simulink model "SecRwLtStFtrstIsPosChk"  (R2024b)
settings: Solver=FixedStepDiscrete  StartTime=0.0  StopTime=10.0  FixedStep=0.01  RelTol=1e-3
undefined symbols (not defined in the file or in its folder): KeSMSuSecRwStFtrstUpwdDnwdPosDelta_Val, KeSMSuSecRwStFtrstUpwdDnwdPosTolr_Val
libraries: StIsPosChkLib x9, simulink x5
settings Model: ModifiedHistory=2023.8.1 V2.0.0 CR401790 增加模式21-26  Creator=sn2xws  LastModifiedBy=sn55gm
settings SolverCC: AlgebraicLoopSolver=TrustRegion
settings DataIOCC: SaveFormat=StructureWithTime  ReturnWorkspaceOutputs=off
settings OptimizationCC: DefaultParameterBehavior=Inlined  EnhancedBackFolding=on  PassReuseOutputArgsAs=Individual arguments  ZeroExternalMemoryAtStartup=off  ZeroInternalMemoryAtStartup=off  OptimizeBlockOrder=speed  DifferentSizesBufferReuse=on  OptimizationCustomize=off  EfficientTunableParamExpr=on
settings DebuggingCC: ParameterTunabilityLossMsg=error  UnconnectedInputMsg=warning  UnconnectedOutputMsg=warning  UnconnectedLineMsg=warning  ArithmeticOperatorsInVariantConditions=warning
settings ModelReferenceCC: EnableRefExpFcnMdlSchedulingChecks=on  ModelReferenceNumInstancesAllowed=Single
settings SFSimCC: MATLABDynamicMemAlloc=off  CustomCodeUndefinedFunction=UseInterfaceOnly
settings RTWCC: Description=AUTOSAR  SystemTargetFile=autosar.tlc  GenCodeOnly=on  TemplateMakefile=ert_default_tmf  GenerateReport=on  IncludeHyperlinkInReport=on  LaunchReport=on  DataTypeReplacement=CDataTypesFixedWidth  GenerateTraceInfo=on  GenerateTraceReport=on  GenerateTraceReportSl=on  GenerateTraceReportSf=on  GenerateTraceReportEml=on  GenerateCodeMetricsReport=on  GPUComputeCapability=3.5
settings CodeAppCC: ForceParamTrailComments=on  IgnoreCustomStorageClasses=off  OperatorAnnotations=on  SimulinkDataObjDesc=on  SFDataObjDesc=on  InsertBlockDesc=on
settings STFCustomTargetCC: TargetLangStandard=C99 (ISO)  MultiwordLength=256  ParMdlRefBuildCompliant=on  CompOptLevelCompliant=on  IncludeMdlTerminateFcn=off  CombineOutputUpdateFcns=on  SuppressErrorStatus=on  ERTCustomFileBanners=on  SupportNonFinite=off  SupportComplex=off  SupportContinuousTime=off  SupportNonInlinedSFcns=off  RemoveResetFunc=on  MATLABClassNameForMDSCustomization=Simulink.SoftwareTarget.ERTCustomization  AutosarCompliant=on  UseToolchainInfoCompliant=on  LookupTableObjectStructAxisOrder=2,1,3,4,...  LUTObjectStructOrderEvenSpacing=Size,Table,Breakpoints  SystemTargetFile=autosar.tlc
settings ERTTargetCC: TargetLangStandard=C99 (ISO)  ConcurrentExecutionCompliant=off  IncludeMdlTerminateFcn=off  SuppressErrorStatus=on  SupportNonFinite=off  SupportComplex=off  ModelStepFunctionPrototypeControlCompliant=off  CPPClassGenCompliant=off  AutosarCompliant=on  LookupTableObjectStructAxisOrder=2,1,3,4,...  LUTObjectStructOrderEvenSpacing=Size,Table,Breakpoints  ERTCustomFileTemplate=example_file_process.tlc  ERTFilePackagingFormat=Compact  BooleanTrueId=TRUE  BooleanFalseId=FALSE  DynamicArrayContainerType=coder::array

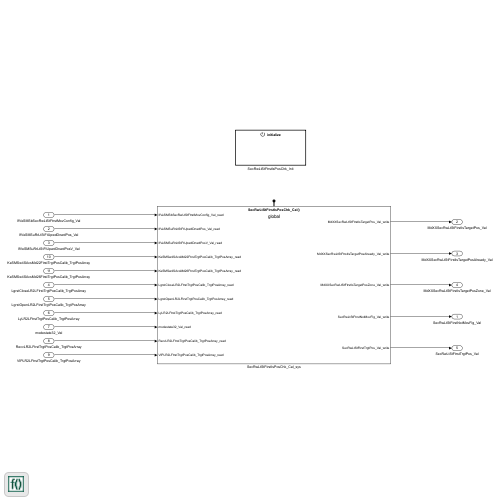
[thumbnail: Simulink's stored preview of the top-level diagram]
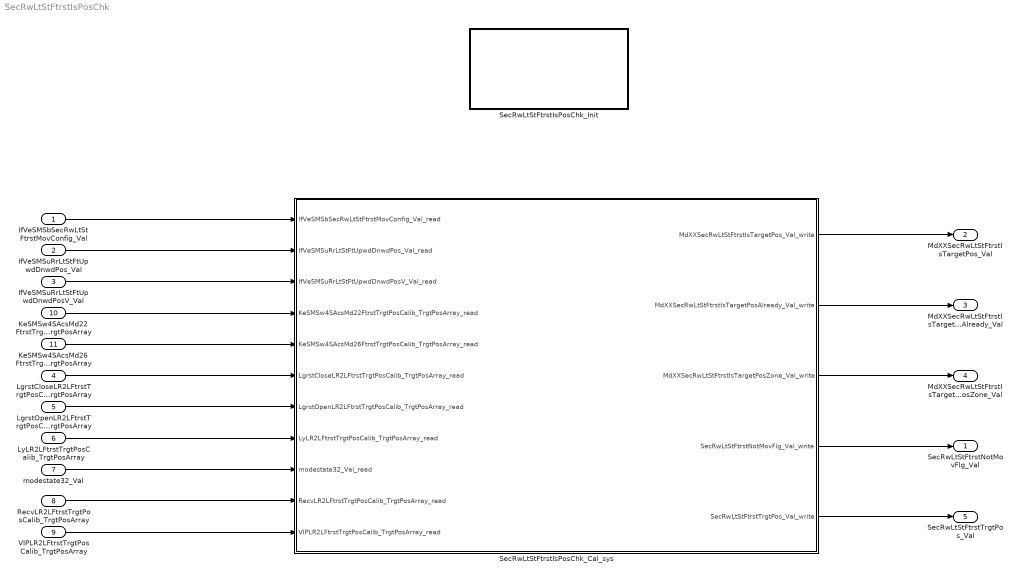
== system SecRwLtStFtrstIsPosChk ==
  IfVeSMSbSecRwLtStFtrstMovConfig_Val : Inport  OutDataTypeStr=boolean  PortDimensions=1
  IfVeSMSuRrLtStFtUpwdDnwdPos_Val : Inport  Port=2  OutDataTypeStr=uint16  PortDimensions=1
  IfVeSMSuRrLtStFtUpwdDnwdPosV_Val : Inport  Port=3  OutDataTypeStr=boolean  PortDimensions=1
  LgrstCloseLR2LFtrstTrgtPosCalib_TrgtPosArray : Inport  Description=|  Port=4  OutDataTypeStr=uint16  PortDimensions=3
      | 0:Pos
      | 1:Max
      | 2:Min
  LgrstOpenLR2LFtrstTrgtPosCalib_TrgtPosArray : Inport  Description=|  Port=5  OutDataTypeStr=uint16  PortDimensions=3
      | 0:Pos
      | 1:Max
      | 2:Min
  LyLR2LFtrstTrgtPosCalib_TrgtPosArray : Inport  Description=|  Port=6  OutDataTypeStr=uint16  PortDimensions=3
      | 0:Pos
      | 1:Max
      | 2:Min
  modestate32_Val : Inport  Port=7  OutDataTypeStr=uint32  PortDimensions=1
  RecvLR2LFtrstTrgtPosCalib_TrgtPosArray : Inport  Description=|  Port=8  OutDataTypeStr=uint16  PortDimensions=3
      | 0:Pos
      | 1:Max
      | 2:Min
  VIPLR2LFtrstTrgtPosCalib_TrgtPosArray : Inport  Description=|  Port=9  OutDataTypeStr=uint16  PortDimensions=3
      | 0:Pos
      | 1:Max
      | 2:Min
  KeSMSw4SAcsMd22FtrstTrgtPosCalib_TrgtPosArray : Inport  Description=|  Port=10  OutDataTypeStr=uint16  PortDimensions=3
      | 0:Pos
      | 1:Max
      | 2:Min
  KeSMSw4SAcsMd26FtrstTrgtPosCalib_TrgtPosArray : Inport  Description=|  Port=11  OutDataTypeStr=uint16  PortDimensions=3
      | 0:Pos
      | 1:Max
      | 2:Min
  SecRwLtStFtrstIsPosChk_Cal_sys : Subsystem
  SecRwLtStFtrstIsPosChk_Init : Subsystem
  SecRwLtStFtrstNotMovFlg_Val : Outport  OutDataTypeStr=boolean  PortDimensions=1  VectorParamsAs1DForOutWhenUnconnected=off
  MdXXSecRwLtStFtrstIsTargetPos_Val : Outport  Port=2  OutDataTypeStr=uint32  PortDimensions=1  VectorParamsAs1DForOutWhenUnconnected=off
  MdXXSecRwLtStFtrstIsTargetPosAlready_Val : Outport  Port=3  OutDataTypeStr=uint32  PortDimensions=1  VectorParamsAs1DForOutWhenUnconnected=off
  MdXXSecRwLtStFtrstIsTargetPosZone_Val : Outport  Port=4  OutDataTypeStr=uint32  PortDimensions=1  VectorParamsAs1DForOutWhenUnconnected=off
  SecRwLtStFtrstTrgtPos_Val : Outport  Port=5  OutDataTypeStr=uint16  PortDimensions=1  VectorParamsAs1DForOutWhenUnconnected=off
  wires:
  IfVeSMSbSecRwLtStFtrstMovConfig_Val/1 -> SecRwLtStFtrstIsPosChk_Cal_sys/1(IfVeSMSbSecRwLtStFtrstMovConfig_Val_read)
  IfVeSMSuRrLtStFtUpwdDnwdPos_Val/1 -> SecRwLtStFtrstIsPosChk_Cal_sys/2(IfVeSMSuRrLtStFtUpwdDnwdPos_Val_read)
  IfVeSMSuRrLtStFtUpwdDnwdPosV_Val/1 -> SecRwLtStFtrstIsPosChk_Cal_sys/3(IfVeSMSuRrLtStFtUpwdDnwdPosV_Val_read)
  LgrstCloseLR2LFtrstTrgtPosCalib_TrgtPosArray/1 -> SecRwLtStFtrstIsPosChk_Cal_sys/6(LgrstCloseLR2LFtrstTrgtPosCalib_TrgtPosArray_read)
  LgrstOpenLR2LFtrstTrgtPosCalib_TrgtPosArray/1 -> SecRwLtStFtrstIsPosChk_Cal_sys/7(LgrstOpenLR2LFtrstTrgtPosCalib_TrgtPosArray_read)
  LyLR2LFtrstTrgtPosCalib_TrgtPosArray/1 -> SecRwLtStFtrstIsPosChk_Cal_sys/8(LyLR2LFtrstTrgtPosCalib_TrgtPosArray_read)
  modestate32_Val/1 -> SecRwLtStFtrstIsPosChk_Cal_sys/9(modestate32_Val_read)
  RecvLR2LFtrstTrgtPosCalib_TrgtPosArray/1 -> SecRwLtStFtrstIsPosChk_Cal_sys/10(RecvLR2LFtrstTrgtPosCalib_TrgtPosArray_read)
  VIPLR2LFtrstTrgtPosCalib_TrgtPosArray/1 -> SecRwLtStFtrstIsPosChk_Cal_sys/11(VIPLR2LFtrstTrgtPosCalib_TrgtPosArray_read)
  SecRwLtStFtrstIsPosChk_Cal_sys/1(MdXXSecRwLtStFtrstIsTargetPos_Val_write) -> MdXXSecRwLtStFtrstIsTargetPos_Val/1
  SecRwLtStFtrstIsPosChk_Cal_sys/2(MdXXSecRwLtStFtrstIsTargetPosAlready_Val_write) -> MdXXSecRwLtStFtrstIsTargetPosAlready_Val/1
  SecRwLtStFtrstIsPosChk_Cal_sys/3(MdXXSecRwLtStFtrstIsTargetPosZone_Val_write) -> MdXXSecRwLtStFtrstIsTargetPosZone_Val/1
  SecRwLtStFtrstIsPosChk_Cal_sys/4(SecRwLtStFtrstNotMovFlg_Val_write) -> SecRwLtStFtrstNotMovFlg_Val/1
  SecRwLtStFtrstIsPosChk_Cal_sys/5(SecRwLtStFtrstTrgtPos_Val_write) -> SecRwLtStFtrstTrgtPos_Val/1
  KeSMSw4SAcsMd22FtrstTrgtPosCalib_TrgtPosArray/1 -> SecRwLtStFtrstIsPosChk_Cal_sys/4(KeSMSw4SAcsMd22FtrstTrgtPosCalib_TrgtPosArray_read)
  KeSMSw4SAcsMd26FtrstTrgtPosCalib_TrgtPosArray/1 -> SecRwLtStFtrstIsPosChk_Cal_sys/5(KeSMSw4SAcsMd26FtrstTrgtPosCalib_TrgtPosArray_read)

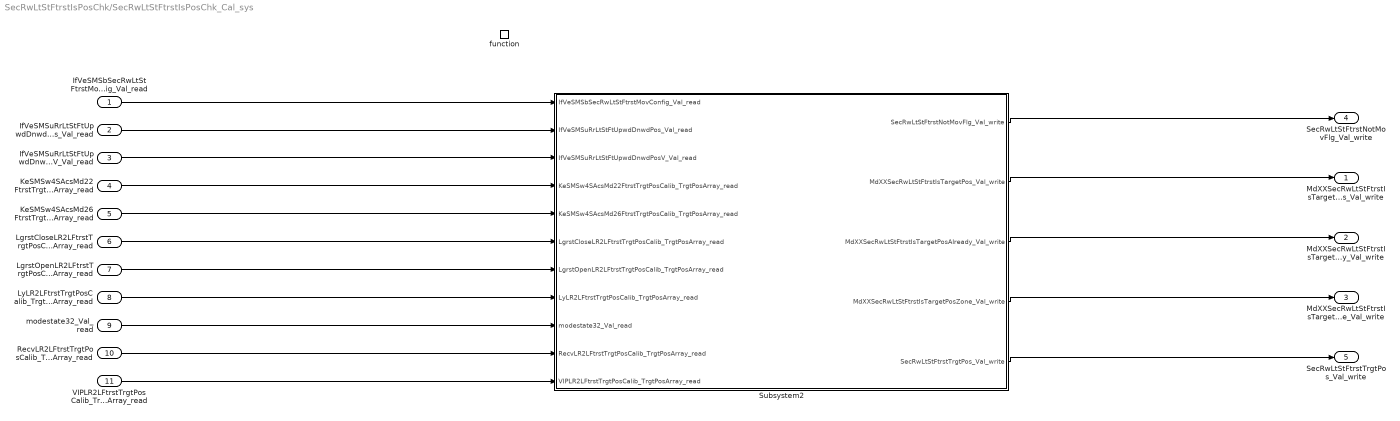
== system SecRwLtStFtrstIsPosChk/SecRwLtStFtrstIsPosChk_Cal_sys ==
  IfVeSMSbSecRwLtStFtrstMovConfig_Val_read : Inport
  IfVeSMSuRrLtStFtUpwdDnwdPos_Val_read : Inport  Port=2
  IfVeSMSuRrLtStFtUpwdDnwdPosV_Val_read : Inport  Port=3
  KeSMSw4SAcsMd22FtrstTrgtPosCalib_TrgtPosArray_read : Inport  Port=4
  KeSMSw4SAcsMd26FtrstTrgtPosCalib_TrgtPosArray_read : Inport  Port=5
  LgrstCloseLR2LFtrstTrgtPosCalib_TrgtPosArray_read : Inport  Port=6
  LgrstOpenLR2LFtrstTrgtPosCalib_TrgtPosArray_read : Inport  Port=7
  LyLR2LFtrstTrgtPosCalib_TrgtPosArray_read : Inport  Port=8
  modestate32_Val_read : Inport  Port=9
  RecvLR2LFtrstTrgtPosCalib_TrgtPosArray_read : Inport  Port=10
  VIPLR2LFtrstTrgtPosCalib_TrgtPosArray_read : Inport  Port=11
  function : TriggerPort  TriggerType=function-call  IsSimulinkFunction=on  FunctionName=SecRwLtStFtrstIsPosChk_Cal  VariantControl=(inherit)
  Subsystem2 : Subsystem
  MdXXSecRwLtStFtrstIsTargetPos_Val_write : Outport  VectorParamsAs1DForOutWhenUnconnected=off
      settings: EnsureOutportIsVirtual=on
  MdXXSecRwLtStFtrstIsTargetPosAlready_Val_write : Outport  Port=2  VectorParamsAs1DForOutWhenUnconnected=off
      settings: EnsureOutportIsVirtual=on
  MdXXSecRwLtStFtrstIsTargetPosZone_Val_write : Outport  Port=3  VectorParamsAs1DForOutWhenUnconnected=off
      settings: EnsureOutportIsVirtual=on
  SecRwLtStFtrstNotMovFlg_Val_write : Outport  Port=4  VectorParamsAs1DForOutWhenUnconnected=off
      settings: EnsureOutportIsVirtual=on
  SecRwLtStFtrstTrgtPos_Val_write : Outport  Port=5  VectorParamsAs1DForOutWhenUnconnected=off
      settings: EnsureOutportIsVirtual=on
  wires:
  Subsystem2/1(SecRwLtStFtrstNotMovFlg_Val_write) -> SecRwLtStFtrstNotMovFlg_Val_write/1
  Subsystem2/2(MdXXSecRwLtStFtrstIsTargetPos_Val_write) -> MdXXSecRwLtStFtrstIsTargetPos_Val_write/1
  Subsystem2/3(MdXXSecRwLtStFtrstIsTargetPosAlready_Val_write) -> MdXXSecRwLtStFtrstIsTargetPosAlready_Val_write/1
  Subsystem2/4(MdXXSecRwLtStFtrstIsTargetPosZone_Val_write) -> MdXXSecRwLtStFtrstIsTargetPosZone_Val_write/1
  Subsystem2/5(SecRwLtStFtrstTrgtPos_Val_write) -> SecRwLtStFtrstTrgtPos_Val_write/1
  IfVeSMSuRrLtStFtUpwdDnwdPos_Val_read/1 -> Subsystem2/2(IfVeSMSuRrLtStFtUpwdDnwdPos_Val_read)
  IfVeSMSbSecRwLtStFtrstMovConfig_Val_read/1 -> Subsystem2/1(IfVeSMSbSecRwLtStFtrstMovConfig_Val_read)
  IfVeSMSuRrLtStFtUpwdDnwdPosV_Val_read/1 -> Subsystem2/3(IfVeSMSuRrLtStFtUpwdDnwdPosV_Val_read)
  KeSMSw4SAcsMd22FtrstTrgtPosCalib_TrgtPosArray_read/1 -> Subsystem2/4(KeSMSw4SAcsMd22FtrstTrgtPosCalib_TrgtPosArray_read)
  KeSMSw4SAcsMd26FtrstTrgtPosCalib_TrgtPosArray_read/1 -> Subsystem2/5(KeSMSw4SAcsMd26FtrstTrgtPosCalib_TrgtPosArray_read)
  LgrstCloseLR2LFtrstTrgtPosCalib_TrgtPosArray_read/1 -> Subsystem2/6(LgrstCloseLR2LFtrstTrgtPosCalib_TrgtPosArray_read)
  LgrstOpenLR2LFtrstTrgtPosCalib_TrgtPosArray_read/1 -> Subsystem2/7(LgrstOpenLR2LFtrstTrgtPosCalib_TrgtPosArray_read)
  LyLR2LFtrstTrgtPosCalib_TrgtPosArray_read/1 -> Subsystem2/8(LyLR2LFtrstTrgtPosCalib_TrgtPosArray_read)
  modestate32_Val_read/1 -> Subsystem2/9(modestate32_Val_read)
  RecvLR2LFtrstTrgtPosCalib_TrgtPosArray_read/1 -> Subsystem2/10(RecvLR2LFtrstTrgtPosCalib_TrgtPosArray_read)
  VIPLR2LFtrstTrgtPosCalib_TrgtPosArray_read/1 -> Subsystem2/11(VIPLR2LFtrstTrgtPosCalib_TrgtPosArray_read)

== system SecRwLtStFtrstIsPosChk/SecRwLtStFtrstIsPosChk_Init ==
  Event Listener : EventListener  EventName=reset

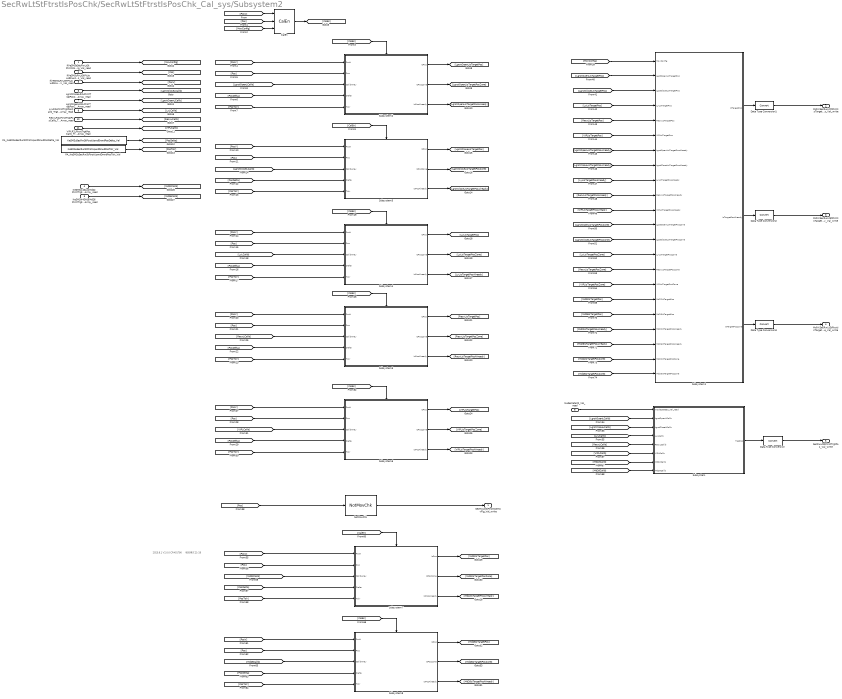
== system SecRwLtStFtrstIsPosChk/SecRwLtStFtrstIsPosChk_Cal_sys/Subsystem2 ==
  note: 2023.8.1 V2.0.0 CR401790 增加模式21-26
  IfVeSMSbSecRwLtStFtrstMovConfig_Val_read : Inport
  IfVeSMSuRrLtStFtUpwdDnwdPos_Val_read : Inport  Port=2
  IfVeSMSuRrLtStFtUpwdDnwdPosV_Val_read : Inport  Port=3
  KeSMSw4SAcsMd22FtrstTrgtPosCalib_TrgtPosArray_read : Inport  Port=4
  KeSMSw4SAcsMd26FtrstTrgtPosCalib_TrgtPosArray_read : Inport  Port=5
  LgrstCloseLR2LFtrstTrgtPosCalib_TrgtPosArray_read : Inport  Port=6
  LgrstOpenLR2LFtrstTrgtPosCalib_TrgtPosArray_read : Inport  Port=7
  LyLR2LFtrstTrgtPosCalib_TrgtPosArray_read : Inport  Port=8
  modestate32_Val_read : Inport  Port=9
  RecvLR2LFtrstTrgtPosCalib_TrgtPosArray_read : Inport  Port=10
  VIPLR2LFtrstTrgtPosCalib_TrgtPosArray_read : Inport  Port=11
  CalEn : StIsPosChkLib/CalEn  SystemSampleTime=-1  VariantActivationTime=update diagram  AllowFlexibleInterface=on  Latency=0  AutoFrameSizeCalculation=off
  Data Type Conversion{,1..3} (4 alike) : DataTypeConversion  SaturateOnIntegerOverflow=off  RndMeth=Floor
  NotMovChk : StIsPosChkLib/NotMovChk  SystemSampleTime=-1  VariantActivationTime=update diagram  AllowFlexibleInterface=on  Latency=0  AutoFrameSizeCalculation=off
  PA_KeSMSuSecRwStFtrstUpwdDnwdPosDelta_Val : Constant  Value=KeSMSuSecRwStFtrstUpwdDnwdPosDelta_Val
  PA_KeSMSuSecRwStFtrstUpwdDnwdPosTolr_Val : Constant  Value=KeSMSuSecRwStFtrstUpwdDnwdPosTolr_Val
  Subsystem : Subsystem
  Subsystem1 : Subsystem
  Subsystem2 : Subsystem
  Subsystem3 : Subsystem
  Subsystem4 : Subsystem
  Subsystem5 : Subsystem
  Subsystem6 : Subsystem
  Subsystem7 : Subsystem
  Subsystem8 : Subsystem
  SecRwLtStFtrstNotMovFlg_Val_write : Outport  VectorParamsAs1DForOutWhenUnconnected=off
      settings: EnsureOutportIsVirtual=on
  MdXXSecRwLtStFtrstIsTargetPos_Val_write : Outport  Port=2  VectorParamsAs1DForOutWhenUnconnected=off
      settings: EnsureOutportIsVirtual=on
  MdXXSecRwLtStFtrstIsTargetPosAlready_Val_write : Outport  Port=3  VectorParamsAs1DForOutWhenUnconnected=off
      settings: EnsureOutportIsVirtual=on
  MdXXSecRwLtStFtrstIsTargetPosZone_Val_write : Outport  Port=4  VectorParamsAs1DForOutWhenUnconnected=off
      settings: EnsureOutportIsVirtual=on
  SecRwLtStFtrstTrgtPos_Val_write : Outport  Port=5  VectorParamsAs1DForOutWhenUnconnected=off
      settings: EnsureOutportIsVirtual=on
  wires:
  [LgrstOpenLIsTargetPosAlready] -> Subsystem1/7(LgrstOpenLIsTargetPosAlready)
  [LgrstOpenLIsTargetPos] -> Subsystem1/2(LgrstOpenLIsTargetPos)
  [LgrstOpenLIsTargetPosZone] -> Subsystem1/12(LgrstOpenLIsTargetPosZone)
  LgrstOpenLR2LFtrstTrgtPosCalib_TrgtPosArray_read/1 -> [LgrstOpenLCalib]
  [Pos] -> Subsystem4/2(Pos)
  NotMovChk/1 -> SecRwLtStFtrstNotMovFlg_Val_write/1
  LyLR2LFtrstTrgtPosCalib_TrgtPosArray_read/1 -> [LyLCalib]
  [LgrstOpenLCalib] -> Subsystem/2(LgrstOpenLCalib)
  VIPLR2LFtrstTrgtPosCalib_TrgtPosArray_read/1 -> [VIPLCalib]
  Subsystem2/2(IsPosZone) -> [LgrstOpenLIsTargetPosZone]
  [PosDelta] -> Subsystem5/4(Delta)
  [PosDelta] -> Subsystem2/4(Delta)
  [Pos] -> Subsystem2/2(Pos)
  [VIPLIsTargetPosAlready] -> Subsystem1/11(VIPLIsTargetPosAlready)
  [PosTolr] -> Subsystem5/5(Tolr)
  [Pos] -> Subsystem6/2(Pos)
  Subsystem3/1(IsPos) -> [LgrstCloseLIsTargetPos]
  PA_KeSMSuSecRwStFtrstUpwdDnwdPosDelta_Val/1 -> [PosDelta]
  Subsystem4/2(IsPosZone) -> [LyLIsTargetPosZone]
  IfVeSMSuRrLtStFtUpwdDnwdPos_Val_read/1 -> [Pos]
  Data Type Conversion2/1 -> MdXXSecRwLtStFtrstIsTargetPosAlready_Val_write/1
  CalEn/1 -> [CalEn]
  IfVeSMSbSecRwLtStFtrstMovConfig_Val_read/1 -> [MovConfig]
  [PosV] -> Subsystem5/1(PosV)
  [CalEn] -> Subsystem2/Enable
  [CalEn] -> Subsystem4/Enable
  [Pos] -> CalEn/2
  [PosTolr] -> Subsystem2/5(Tolr)
  [VIPLCalib] -> Subsystem/6(VIPLCalib)
  Subsystem2/3(IsPosAlready) -> [LgrstOpenLIsTargetPosAlready]
  [PosTolr] -> Subsystem3/5(Tolr)
  [PosTolr] -> Subsystem6/5(Tolr)
  [Pos] -> NotMovChk/1
  [LgrstCloseLIsTargetPos] -> Subsystem1/3(LgrstCloseLIsTargetPos)
  Subsystem6/3(IsPosAlready) -> [VIPLIsTargetPosAlready]
  Subsystem2/1(IsPos) -> [LgrstOpenLIsTargetPos]
  [PosV] -> Subsystem3/1(PosV)
  Subsystem5/3(IsPosAlready) -> [RecvLIsTargetPosAlready]
  Subsystem5/1(IsPos) -> [RecvLIsTargetPos]
  [VIPLCalib] -> Subsystem6/3(CalibArray)
  [LyLCalib] -> Subsystem4/3(CalibArray)
  RecvLR2LFtrstTrgtPosCalib_TrgtPosArray_read/1 -> [RecvLCalib]
  [Pos] -> Subsystem3/2(Pos)
  [LyLIsTargetPos] -> Subsystem1/4(LyLIsTargetPos)
  [MovConfig] -> CalEn/3
  Subsystem4/1(IsPos) -> [LyLIsTargetPos]
  [LyLIsTargetPosAlready] -> Subsystem1/9(LyLIsTargetPosAlready)
  Subsystem3/2(IsPosZone) -> [LgrstCloseLIsTargetPosZone]
  Subsystem6/1(IsPos) -> [VIPLIsTargetPos]
  Subsystem1/2(IsTargetPosAlready) -> Data Type Conversion2/1
  [VIPLIsTargetPosZone] -> Subsystem1/16(VIPLIsTargetPosZone)
  [CalEn] -> Subsystem5/Enable
  [PosV] -> CalEn/1
  Subsystem4/3(IsPosAlready) -> [LyLIsTargetPosAlready]
  [RecvLCalib] -> Subsystem/5(RecvLCalib)
  Subsystem5/2(IsPosZone) -> [RecvLIsTargetPosZone]
  [RecvLCalib] -> Subsystem5/3(CalibArray)
  Subsystem3/3(IsPosAlready) -> [LgrstCloseLIsTargetPosAlready]
  [PosV] -> Subsystem2/1(PosV)
  [VIPLIsTargetPos] -> Subsystem1/6(VIPLIsTargetPos)
  [PosV] -> Subsystem6/1(PosV)
  [LyLCalib] -> Subsystem/4(LyLCalib)
  modestate32_Val_read/1 -> Subsystem/1(modestate32_Val_read)
  [LyLIsTargetPosZone] -> Subsystem1/14(LyLIsTargetPosZone)
  [LgrstCloseLIsTargetPosZone] -> Subsystem1/13(LgrstCloseLIsTargetPosZone)
  PA_KeSMSuSecRwStFtrstUpwdDnwdPosTolr_Val/1 -> [PosTolr]
  [RecvLIsTargetPos] -> Subsystem1/5(RecvLIsTargetPos)
  [CalEn] -> Subsystem3/Enable
  [MovConfig] -> Subsystem1/1(MovConfig)
  [RecvLIsTargetPosZone] -> Subsystem1/15(RecvLIsTargetPosZone)
  [Pos] -> Subsystem5/2(Pos)
  [LgrstCloseLIsTargetPosAlready] -> Subsystem1/8(LgrstCloseLIsTargetPosAlready)
  [LgrstCloseLCalib] -> Subsystem/3(LgrstCloseLCalib)
  [PosDelta] -> Subsystem4/4(Delta)
  Subsystem/1(TrgtPos) -> Data Type Conversion/1
  [PosDelta] -> Subsystem3/4(Delta)
  [CalEn] -> Subsystem6/Enable
  LgrstCloseLR2LFtrstTrgtPosCalib_TrgtPosArray_read/1 -> [LgrstCloseLCalib]
  [PosTolr] -> Subsystem4/5(Tolr)
  [RecvLIsTargetPosAlready] -> Subsystem1/10(RecvLIsTargetPosAlready)
  IfVeSMSuRrLtStFtUpwdDnwdPosV_Val_read/1 -> [PosV]
  [PosV] -> Subsystem4/1(PosV)
  Data Type Conversion1/1 -> MdXXSecRwLtStFtrstIsTargetPos_Val_write/1
  [PosDelta] -> Subsystem6/4(Delta)
  Subsystem1/3(IsTargetPosZone) -> Data Type Conversion3/1
  Data Type Conversion3/1 -> MdXXSecRwLtStFtrstIsTargetPosZone_Val_write/1
  Subsystem1/1(IsTargetPos) -> Data Type Conversion1/1
  Data Type Conversion/1 -> SecRwLtStFtrstTrgtPos_Val_write/1
  Subsystem6/2(IsPosZone) -> [VIPLIsTargetPosZone]
  KeSMSw4SAcsMd22FtrstTrgtPosCalib_TrgtPosArray_read/1 -> [Md22Calib]
  KeSMSw4SAcsMd26FtrstTrgtPosCalib_TrgtPosArray_read/1 -> [Md26Calib]
  Subsystem7/2(IsPosZone) -> [Md22IsTargetPosZone]
  [PosDelta] -> Subsystem7/4(Delta)
  [CalEn] -> Subsystem7/Enable
  [PosV] -> Subsystem7/1(PosV)
  Subsystem7/1(IsPos) -> [Md22IsTargetPos]
  [Md22Calib] -> Subsystem7/3(CalibArray)
  Subsystem7/3(IsPosAlready) -> [Md22IsTargetPosAlready]
  [PosTolr] -> Subsystem7/5(Tolr)
  [Pos] -> Subsystem7/2(Pos)
  [Pos] -> Subsystem8/2(Pos)
  [PosTolr] -> Subsystem8/5(Tolr)
  Subsystem8/3(IsPosAlready) -> [Md26IsTargetPosAlready]
  [Md26Calib] -> Subsystem8/3(CalibArray)
  Subsystem8/1(IsPos) -> [Md26IsTargetPos]
  [PosV] -> Subsystem8/1(PosV)
  [CalEn] -> Subsystem8/Enable
  [PosDelta] -> Subsystem8/4(Delta)
  Subsystem8/2(IsPosZone) -> [Md26IsTargetPosZone]
  [Md22Calib] -> Subsystem/7(Md22Calib)
  [Md26Calib] -> Subsystem/8(Md26Calib)
  [Md22IsTargetPos] -> Subsystem1/17(Md22IsTargetPos)
  [Md26IsTargetPos] -> Subsystem1/18(Md26IsTargetPos)
  [Md22IsTargetPosAlready] -> Subsystem1/19(Md22IsTargetPosAlready)
  [Md26IsTargetPosAlready] -> Subsystem1/20(Md26IsTargetPosAlready)
  [Md26IsTargetPosZone] -> Subsystem1/22(Md26IsTargetPosZone)
  [Md22IsTargetPosZone] -> Subsystem1/21(Md22IsTargetPosZone)
  [LgrstOpenLCalib] -> Subsystem2/3(CalibArray)
  [LgrstCloseLCalib] -> Subsystem3/3(CalibArray)

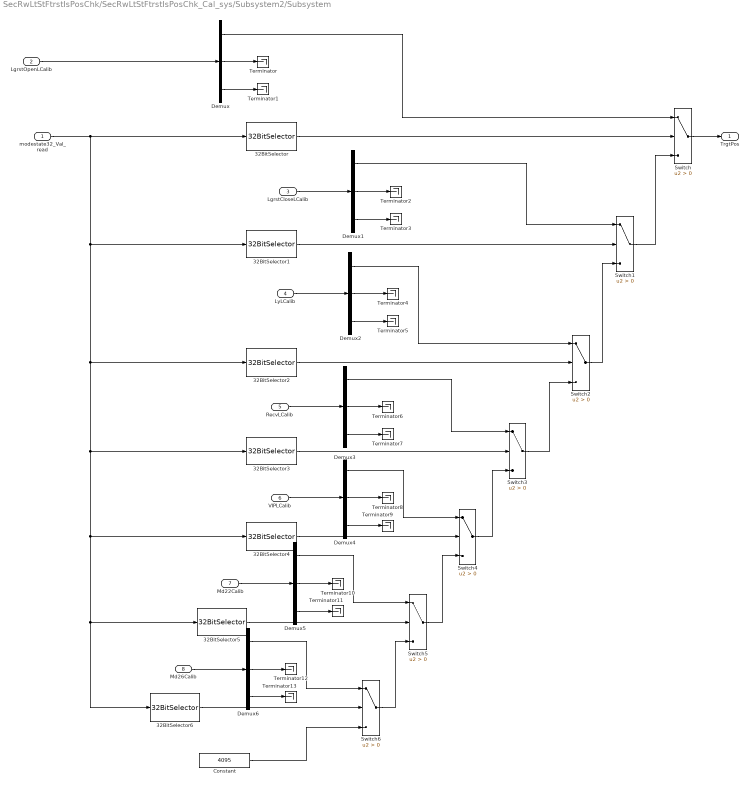
== system SecRwLtStFtrstIsPosChk/SecRwLtStFtrstIsPosChk_Cal_sys/Subsystem2/Subsystem ==
  modestate32_Val_read : Inport
  LgrstOpenLCalib : Inport  Port=2
  LgrstCloseLCalib : Inport  Port=3
  LyLCalib : Inport  Port=4
  RecvLCalib : Inport  Port=5
  VIPLCalib : Inport  Port=6
  Md22Calib : Inport  Port=7
  Md26Calib : Inport  Port=8
  32BitSelector : StIsPosChkLib/32BitSelector  BitNum=15
  32BitSelector1 : StIsPosChkLib/32BitSelector  BitNum=16
  32BitSelector2 : StIsPosChkLib/32BitSelector  BitNum=13
  32BitSelector3 : StIsPosChkLib/32BitSelector  BitNum=10
  32BitSelector4 : StIsPosChkLib/32BitSelector  BitNum=9
  32BitSelector5 : StIsPosChkLib/32BitSelector  BitNum=21
  32BitSelector6 : StIsPosChkLib/32BitSelector  BitNum=25
  Constant : Constant  Value=4095  OutDataTypeStr=uint16
  Demux{,1..6} (7 alike) : Demux  Outputs=3
  Switch{,1..6} (7 alike) : Switch  Criteria=u2 > Threshold  SaturateOnIntegerOverflow=off  InputSameDT=off
  Terminator{,1..13} (14 alike) : Terminator
  TrgtPos : Outport  VectorParamsAs1DForOutWhenUnconnected=off
      settings: EnsureOutportIsVirtual=on
  wires:
  32BitSelector/1 -> Switch/2
  Demux/1 -> Switch/1
  Demux/3 -> Terminator1/1
  Demux/2 -> Terminator/1
  LgrstOpenLCalib/1 -> Demux/1
  LgrstCloseLCalib/1 -> Demux1/1
  Demux1/2 -> Terminator2/1
  Demux1/3 -> Terminator3/1
  Demux1/1 -> Switch1/1
  Switch/1 -> TrgtPos/1
  Switch1/1 -> Switch/3
  32BitSelector1/1 -> Switch1/2
  Switch2/1 -> Switch1/3
  Switch3/1 -> Switch2/3
  Switch4/1 -> Switch3/3
  32BitSelector2/1 -> Switch2/2
  32BitSelector3/1 -> Switch3/2
  32BitSelector4/1 -> Switch4/2
  Demux2/1 -> Switch2/1
  Demux2/3 -> Terminator5/1
  Demux2/2 -> Terminator4/1
  LyLCalib/1 -> Demux2/1
  RecvLCalib/1 -> Demux3/1
  Demux3/2 -> Terminator6/1
  Demux3/3 -> Terminator7/1
  Demux3/1 -> Switch3/1
  Demux4/1 -> Switch4/1
  Demux4/3 -> Terminator9/1
  Demux4/2 -> Terminator8/1
  VIPLCalib/1 -> Demux4/1
  Md22Calib/1 -> Demux5/1
  Demux5/2 -> Terminator10/1
  Demux5/3 -> Terminator11/1
  Demux5/1 -> Switch5/1
  32BitSelector5/1 -> Switch5/2
  Switch5/1 -> Switch4/3
  modestate32_Val_read/1 -> 32BitSelector/1, 32BitSelector1/1, 32BitSelector2/1, 32BitSelector3/1, 32BitSelector6/1, 32BitSelector5/1, 32BitSelector4/1
  Switch6/1 -> Switch5/3
  32BitSelector6/1 -> Switch6/2
  Demux6/1 -> Switch6/1
  Demux6/3 -> Terminator13/1
  Demux6/2 -> Terminator12/1
  Md26Calib/1 -> Demux6/1
  Constant/1 -> Switch6/3

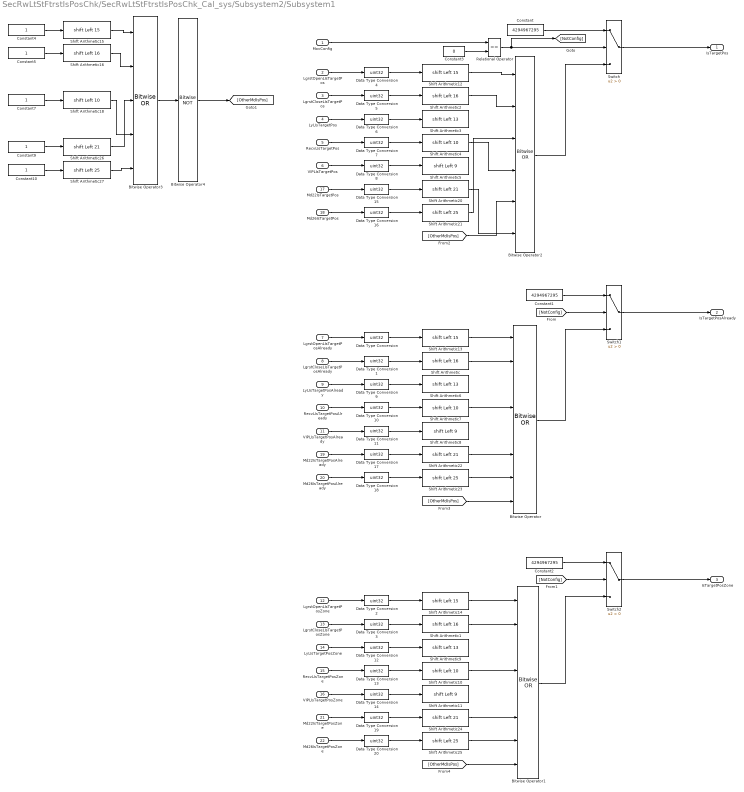
== system SecRwLtStFtrstIsPosChk/SecRwLtStFtrstIsPosChk_Cal_sys/Subsystem2/Subsystem1 ==
  MovConfig : Inport
  LgrstOpenLIsTargetPos : Inport  Port=2
  LgrstCloseLIsTargetPos : Inport  Port=3
  LyLIsTargetPos : Inport  Port=4
  RecvLIsTargetPos : Inport  Port=5
  VIPLIsTargetPos : Inport  Port=6
  LgrstOpenLIsTargetPosAlready : Inport  Port=7
  LgrstCloseLIsTargetPosAlready : Inport  Port=8
  LyLIsTargetPosAlready : Inport  Port=9
  RecvLIsTargetPosAlready : Inport  Port=10
  VIPLIsTargetPosAlready : Inport  Port=11
  LgrstOpenLIsTargetPosZone : Inport  Port=12
  LgrstCloseLIsTargetPosZone : Inport  Port=13
  LyLIsTargetPosZone : Inport  Port=14
  RecvLIsTargetPosZone : Inport  Port=15
  VIPLIsTargetPosZone : Inport  Port=16
  Md22IsTargetPos : Inport  Port=17
  Md26IsTargetPos : Inport  Port=18
  Md22IsTargetPosAlready : Inport  Port=19
  Md26IsTargetPosAlready : Inport  Port=20
  Md22IsTargetPosZone : Inport  Port=21
  Md26IsTargetPosZone : Inport  Port=22
  Bitwise Operator : simulink/Logic and Bit Operations/Bitwise Operator  logicop=OR  UseBitMask=off  NumInputPorts=8  BitMask=bin2dec('11011001')  BitMaskRealWorld=Stored Integer
  Bitwise Operator1 : simulink/Logic and Bit Operations/Bitwise Operator  logicop=OR  UseBitMask=off  NumInputPorts=8  BitMask=bin2dec('11011001')  BitMaskRealWorld=Stored Integer
  Bitwise Operator2 : simulink/Logic and Bit Operations/Bitwise Operator  logicop=OR  UseBitMask=off  NumInputPorts=6  BitMask=bin2dec('11011001')  BitMaskRealWorld=Stored Integer
  Bitwise Operator3 : simulink/Logic and Bit Operations/Bitwise Operator  logicop=OR  UseBitMask=off  NumInputPorts=5  BitMask=bin2dec('11011001')  BitMaskRealWorld=Stored Integer
  Bitwise Operator4 : simulink/Logic and Bit Operations/Bitwise Operator  logicop=NOT  UseBitMask=off  BitMask=bin2dec('11011001')  BitMaskRealWorld=Stored Integer
  Constant : Constant  Value=4294967295  OutDataTypeStr=uint32
  Constant1 : Constant  Value=4294967295  OutDataTypeStr=uint32
  Constant{4..5,7,9..10} (5 alike) : Constant  OutDataTypeStr=uint32
  Constant2 : Constant  Value=4294967295  OutDataTypeStr=uint32
  Constant3 : Constant  Value=0  OutDataTypeStr=uint8
  Data Type Conversion{,1..20} (21 alike) : DataTypeConversion  OutDataTypeStr=uint32  SaturateOnIntegerOverflow=off  RndMeth=Floor
  Relational Operator : RelationalOperator  Operator===  OutDataTypeStr=boolean  RndMeth=Simplest  InputSameDT=off
  Shift Arithmetic{,1..2,16} (4 alike) : ArithShift  BitShiftNumber=16  BitShiftDirection=Left
  Shift Arithmetic{4,7,10,18} (4 alike) : ArithShift  BitShiftNumber=10  BitShiftDirection=Left
  Shift Arithmetic11 : ArithShift  BitShiftNumber=9  BitShiftDirection=Left
  Shift Arithmetic{12..15} (4 alike) : ArithShift  BitShiftNumber=15  BitShiftDirection=Left
  Shift Arithmetic{20,22,24,26} (4 alike) : ArithShift  BitShiftNumber=21  BitShiftDirection=Left
  Shift Arithmetic{21,23,25,27} (4 alike) : ArithShift  BitShiftNumber=25  BitShiftDirection=Left
  Shift Arithmetic3 : ArithShift  BitShiftNumber=13  BitShiftDirection=Left
  Shift Arithmetic5 : ArithShift  BitShiftNumber=9  BitShiftDirection=Left
  Shift Arithmetic6 : ArithShift  BitShiftNumber=13  BitShiftDirection=Left
  Shift Arithmetic8 : ArithShift  BitShiftNumber=9  BitShiftDirection=Left
  Shift Arithmetic9 : ArithShift  BitShiftNumber=13  BitShiftDirection=Left
  Switch : Switch  Criteria=u2 > Threshold  SaturateOnIntegerOverflow=off  InputSameDT=off
  Switch1 : Switch  Criteria=u2 > Threshold  SaturateOnIntegerOverflow=off  InputSameDT=off
  Switch2 : Switch  Criteria=u2 > Threshold  SaturateOnIntegerOverflow=off  InputSameDT=off
  IsTargetPos : Outport  VectorParamsAs1DForOutWhenUnconnected=off
      settings: EnsureOutportIsVirtual=on
  IsTargetPosAlready : Outport  Port=2  VectorParamsAs1DForOutWhenUnconnected=off
      settings: EnsureOutportIsVirtual=on
  IsTargetPosZone : Outport  Port=3  VectorParamsAs1DForOutWhenUnconnected=off
      settings: EnsureOutportIsVirtual=on
  wires:
  Constant3/1 -> Relational Operator/2
  Constant/1 -> Switch/1
  Relational Operator/1 -> [NotConfig], Switch/2
  MovConfig/1 -> Relational Operator/1
  Switch/1 -> IsTargetPos/1
  [NotConfig] -> Switch1/2
  Constant1/1 -> Switch1/1
  Switch1/1 -> IsTargetPosAlready/1
  Switch2/1 -> IsTargetPosZone/1
  Constant2/1 -> Switch2/1
  [NotConfig] -> Switch2/2
  Data Type Conversion1/1 -> Shift Arithmetic/1
  Data Type Conversion/1 -> Shift Arithmetic13/1
  Shift Arithmetic/1 -> Bitwise Operator/2
  Shift Arithmetic1/1 -> Bitwise Operator1/2
  Data Type Conversion2/1 -> Shift Arithmetic14/1
  Data Type Conversion3/1 -> Shift Arithmetic1/1
  Bitwise Operator1/1 -> Switch2/3
  Bitwise Operator/1 -> Switch1/3
  Shift Arithmetic2/1 -> Bitwise Operator2/2
  Data Type Conversion4/1 -> Shift Arithmetic12/1
  Data Type Conversion5/1 -> Shift Arithmetic2/1
  Bitwise Operator2/1 -> Switch/3
  LgrstOpenLIsTargetPos/1 -> Data Type Conversion4/1
  LgrstCloseLIsTargetPos/1 -> Data Type Conversion5/1
  LgrstCloseLIsTargetPosZone/1 -> Data Type Conversion3/1
  LgrstOpenLIsTargetPosZone/1 -> Data Type Conversion2/1
  LgrstCloseLIsTargetPosAlready/1 -> Data Type Conversion1/1
  LgrstOpenLIsTargetPosAlready/1 -> Data Type Conversion/1
  Shift Arithmetic4/1 -> Bitwise Operator2/4
  Data Type Conversion7/1 -> Shift Arithmetic4/1
  Data Type Conversion6/1 -> Shift Arithmetic3/1
  Data Type Conversion8/1 -> Shift Arithmetic5/1
  LyLIsTargetPos/1 -> Data Type Conversion6/1
  RecvLIsTargetPos/1 -> Data Type Conversion7/1
  VIPLIsTargetPos/1 -> Data Type Conversion8/1
  VIPLIsTargetPosAlready/1 -> Data Type Conversion11/1
  RecvLIsTargetPosAlready/1 -> Data Type Conversion10/1
  LyLIsTargetPosAlready/1 -> Data Type Conversion9/1
  Data Type Conversion11/1 -> Shift Arithmetic8/1
  Data Type Conversion9/1 -> Shift Arithmetic6/1
  Data Type Conversion10/1 -> Shift Arithmetic7/1
  Shift Arithmetic7/1 -> Bitwise Operator/4
  Data Type Conversion14/1 -> Shift Arithmetic11/1
  Data Type Conversion13/1 -> Shift Arithmetic10/1
  VIPLIsTargetPosZone/1 -> Data Type Conversion14/1
  Shift Arithmetic10/1 -> Bitwise Operator1/4
  RecvLIsTargetPosZone/1 -> Data Type Conversion13/1
  LyLIsTargetPosZone/1 -> Data Type Conversion12/1
  Data Type Conversion12/1 -> Shift Arithmetic9/1
  Shift Arithmetic12/1 -> Bitwise Operator2/1
  Shift Arithmetic13/1 -> Bitwise Operator/1
  Shift Arithmetic14/1 -> Bitwise Operator1/1
  Constant4/1 -> Shift Arithmetic15/1
  Constant5/1 -> Shift Arithmetic16/1
  Constant7/1 -> Shift Arithmetic18/1
  Shift Arithmetic15/1 -> Bitwise Operator3/1
  Shift Arithmetic16/1 -> Bitwise Operator3/2
  Shift Arithmetic18/1 -> Bitwise Operator3/4
  Bitwise Operator3/1 -> Bitwise Operator4/1
  Bitwise Operator4/1 -> [OtherMdIsPos]
  [OtherMdIsPos] -> Bitwise Operator2/5
  Data Type Conversion15/1 -> Shift Arithmetic20/1
  Shift Arithmetic20/1 -> Bitwise Operator2/6
  Md22IsTargetPos/1 -> Data Type Conversion15/1
  Md26IsTargetPos/1 -> Data Type Conversion16/1
  Shift Arithmetic21/1 -> Bitwise Operator2/3
  Data Type Conversion16/1 -> Shift Arithmetic21/1
  [OtherMdIsPos] -> Bitwise Operator/8
  [OtherMdIsPos] -> Bitwise Operator1/8
  Data Type Conversion18/1 -> Shift Arithmetic23/1
  Shift Arithmetic23/1 -> Bitwise Operator/7
  Md26IsTargetPosAlready/1 -> Data Type Conversion18/1
  Md22IsTargetPosAlready/1 -> Data Type Conversion17/1
  Shift Arithmetic22/1 -> Bitwise Operator/6
  Data Type Conversion17/1 -> Shift Arithmetic22/1
  Data Type Conversion19/1 -> Shift Arithmetic24/1
  Shift Arithmetic24/1 -> Bitwise Operator1/6
  Md22IsTargetPosZone/1 -> Data Type Conversion19/1
  Md26IsTargetPosZone/1 -> Data Type Conversion20/1
  Shift Arithmetic25/1 -> Bitwise Operator1/7
  Data Type Conversion20/1 -> Shift Arithmetic25/1
  Constant9/1 -> Shift Arithmetic26/1
  Shift Arithmetic26/1 -> Bitwise Operator3/3
  Shift Arithmetic27/1 -> Bitwise Operator3/5
  Constant10/1 -> Shift Arithmetic27/1

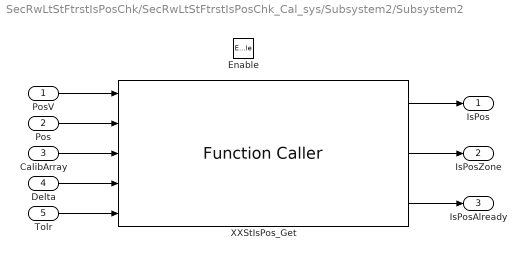
== system SecRwLtStFtrstIsPosChk/SecRwLtStFtrstIsPosChk_Cal_sys/Subsystem2/Subsystem2 ==
  PosV : Inport
  Pos : Inport  Port=2
  CalibArray : Inport  Port=3
  Delta : Inport  Port=4
  Tolr : Inport  Port=5
  Enable : EnablePort
  XXStIsPos_Get : FunctionCaller  FunctionPrototype=[IsPos,IsPosZone,IsPosAlready] = XXStIsPos_Get(PosV,Pos,CalibArray,Delta,Tolr)  InputArgumentSpecifications=boolean(true), uint16(1), uint16([1;1;1]), uint16(1), uint16(1)  OutputArgumentSpecifications=boolean(true), boolean(true), boolean(true)
  IsPos : Outport  VectorParamsAs1DForOutWhenUnconnected=off
  IsPosZone : Outport  Port=2  VectorParamsAs1DForOutWhenUnconnected=off
  IsPosAlready : Outport  Port=3  VectorParamsAs1DForOutWhenUnconnected=off
  wires:
  Delta/1 -> XXStIsPos_Get/4
  CalibArray/1 -> XXStIsPos_Get/3
  Tolr/1 -> XXStIsPos_Get/5
  PosV/1 -> XXStIsPos_Get/1
  XXStIsPos_Get/2 -> IsPosZone/1
  XXStIsPos_Get/3 -> IsPosAlready/1
  Pos/1 -> XXStIsPos_Get/2
  XXStIsPos_Get/1 -> IsPos/1

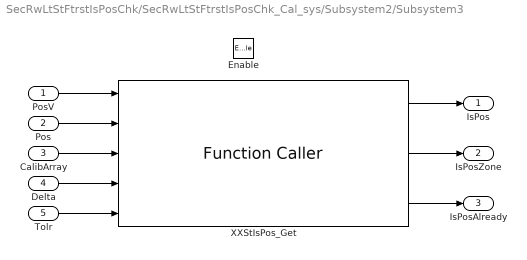
== system SecRwLtStFtrstIsPosChk/SecRwLtStFtrstIsPosChk_Cal_sys/Subsystem2/Subsystem3 ==
  PosV : Inport
  Pos : Inport  Port=2
  CalibArray : Inport  Port=3
  Delta : Inport  Port=4
  Tolr : Inport  Port=5
  Enable : EnablePort
  XXStIsPos_Get : FunctionCaller  FunctionPrototype=[IsPos,IsPosZone,IsPosAlready] = XXStIsPos_Get(PosV,Pos,CalibArray,Delta,Tolr)  InputArgumentSpecifications=boolean(true), uint16(1), uint16([1;1;1]), uint16(1), uint16(1)  OutputArgumentSpecifications=boolean(true), boolean(true), boolean(true)
  IsPos : Outport  VectorParamsAs1DForOutWhenUnconnected=off
  IsPosZone : Outport  Port=2  VectorParamsAs1DForOutWhenUnconnected=off
  IsPosAlready : Outport  Port=3  VectorParamsAs1DForOutWhenUnconnected=off
  wires:
  Delta/1 -> XXStIsPos_Get/4
  CalibArray/1 -> XXStIsPos_Get/3
  Tolr/1 -> XXStIsPos_Get/5
  PosV/1 -> XXStIsPos_Get/1
  XXStIsPos_Get/2 -> IsPosZone/1
  XXStIsPos_Get/3 -> IsPosAlready/1
  Pos/1 -> XXStIsPos_Get/2
  XXStIsPos_Get/1 -> IsPos/1

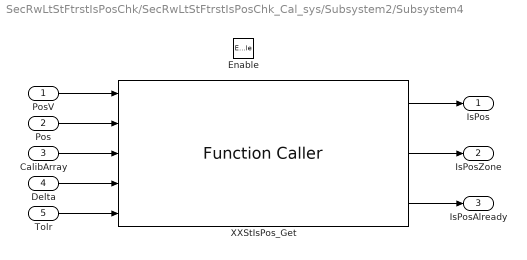
== system SecRwLtStFtrstIsPosChk/SecRwLtStFtrstIsPosChk_Cal_sys/Subsystem2/Subsystem4 ==
  PosV : Inport
  Pos : Inport  Port=2
  CalibArray : Inport  Port=3
  Delta : Inport  Port=4
  Tolr : Inport  Port=5
  Enable : EnablePort
  XXStIsPos_Get : FunctionCaller  FunctionPrototype=[IsPos,IsPosZone,IsPosAlready] = XXStIsPos_Get(PosV,Pos,CalibArray,Delta,Tolr)  InputArgumentSpecifications=boolean(true), uint16(1), uint16([1;1;1]), uint16(1), uint16(1)  OutputArgumentSpecifications=boolean(true), boolean(true), boolean(true)
  IsPos : Outport  VectorParamsAs1DForOutWhenUnconnected=off
  IsPosZone : Outport  Port=2  VectorParamsAs1DForOutWhenUnconnected=off
  IsPosAlready : Outport  Port=3  VectorParamsAs1DForOutWhenUnconnected=off
  wires:
  Delta/1 -> XXStIsPos_Get/4
  CalibArray/1 -> XXStIsPos_Get/3
  Tolr/1 -> XXStIsPos_Get/5
  PosV/1 -> XXStIsPos_Get/1
  XXStIsPos_Get/2 -> IsPosZone/1
  XXStIsPos_Get/3 -> IsPosAlready/1
  Pos/1 -> XXStIsPos_Get/2
  XXStIsPos_Get/1 -> IsPos/1

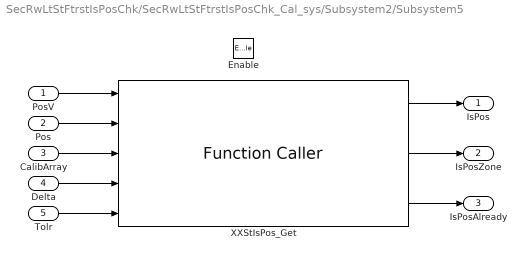
== system SecRwLtStFtrstIsPosChk/SecRwLtStFtrstIsPosChk_Cal_sys/Subsystem2/Subsystem5 ==
  PosV : Inport
  Pos : Inport  Port=2
  CalibArray : Inport  Port=3
  Delta : Inport  Port=4
  Tolr : Inport  Port=5
  Enable : EnablePort
  XXStIsPos_Get : FunctionCaller  FunctionPrototype=[IsPos,IsPosZone,IsPosAlready] = XXStIsPos_Get(PosV,Pos,CalibArray,Delta,Tolr)  InputArgumentSpecifications=boolean(true), uint16(1), uint16([1;1;1]), uint16(1), uint16(1)  OutputArgumentSpecifications=boolean(true), boolean(true), boolean(true)
  IsPos : Outport  VectorParamsAs1DForOutWhenUnconnected=off
  IsPosZone : Outport  Port=2  VectorParamsAs1DForOutWhenUnconnected=off
  IsPosAlready : Outport  Port=3  VectorParamsAs1DForOutWhenUnconnected=off
  wires:
  Delta/1 -> XXStIsPos_Get/4
  CalibArray/1 -> XXStIsPos_Get/3
  Tolr/1 -> XXStIsPos_Get/5
  PosV/1 -> XXStIsPos_Get/1
  XXStIsPos_Get/2 -> IsPosZone/1
  XXStIsPos_Get/3 -> IsPosAlready/1
  Pos/1 -> XXStIsPos_Get/2
  XXStIsPos_Get/1 -> IsPos/1

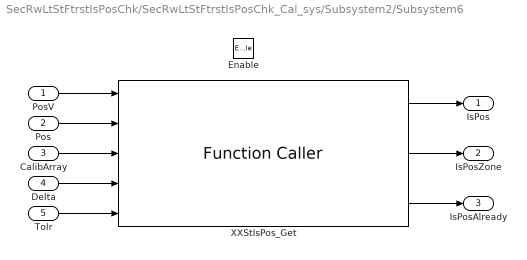
== system SecRwLtStFtrstIsPosChk/SecRwLtStFtrstIsPosChk_Cal_sys/Subsystem2/Subsystem6 ==
  PosV : Inport
  Pos : Inport  Port=2
  CalibArray : Inport  Port=3
  Delta : Inport  Port=4
  Tolr : Inport  Port=5
  Enable : EnablePort
  XXStIsPos_Get : FunctionCaller  FunctionPrototype=[IsPos,IsPosZone,IsPosAlready] = XXStIsPos_Get(PosV,Pos,CalibArray,Delta,Tolr)  InputArgumentSpecifications=boolean(true), uint16(1), uint16([1;1;1]), uint16(1), uint16(1)  OutputArgumentSpecifications=boolean(true), boolean(true), boolean(true)
  IsPos : Outport  VectorParamsAs1DForOutWhenUnconnected=off
  IsPosZone : Outport  Port=2  VectorParamsAs1DForOutWhenUnconnected=off
  IsPosAlready : Outport  Port=3  VectorParamsAs1DForOutWhenUnconnected=off
  wires:
  Delta/1 -> XXStIsPos_Get/4
  CalibArray/1 -> XXStIsPos_Get/3
  Tolr/1 -> XXStIsPos_Get/5
  PosV/1 -> XXStIsPos_Get/1
  XXStIsPos_Get/2 -> IsPosZone/1
  XXStIsPos_Get/3 -> IsPosAlready/1
  Pos/1 -> XXStIsPos_Get/2
  XXStIsPos_Get/1 -> IsPos/1

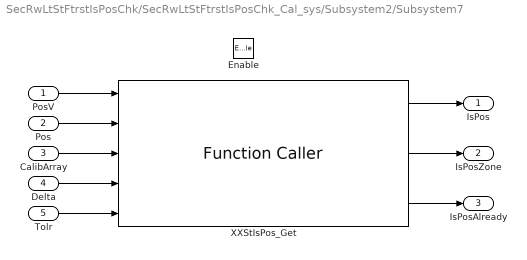
== system SecRwLtStFtrstIsPosChk/SecRwLtStFtrstIsPosChk_Cal_sys/Subsystem2/Subsystem7 ==
  PosV : Inport
  Pos : Inport  Port=2
  CalibArray : Inport  Port=3
  Delta : Inport  Port=4
  Tolr : Inport  Port=5
  Enable : EnablePort
  XXStIsPos_Get : FunctionCaller  FunctionPrototype=[IsPos,IsPosZone,IsPosAlready] = XXStIsPos_Get(PosV,Pos,CalibArray,Delta,Tolr)  InputArgumentSpecifications=boolean(true), uint16(1), uint16([1;1;1]), uint16(1), uint16(1)  OutputArgumentSpecifications=boolean(true), boolean(true), boolean(true)
  IsPos : Outport  VectorParamsAs1DForOutWhenUnconnected=off
  IsPosZone : Outport  Port=2  VectorParamsAs1DForOutWhenUnconnected=off
  IsPosAlready : Outport  Port=3  VectorParamsAs1DForOutWhenUnconnected=off
  wires:
  XXStIsPos_Get/1 -> IsPos/1
  Pos/1 -> XXStIsPos_Get/2
  XXStIsPos_Get/3 -> IsPosAlready/1
  XXStIsPos_Get/2 -> IsPosZone/1
  PosV/1 -> XXStIsPos_Get/1
  Tolr/1 -> XXStIsPos_Get/5
  CalibArray/1 -> XXStIsPos_Get/3
  Delta/1 -> XXStIsPos_Get/4

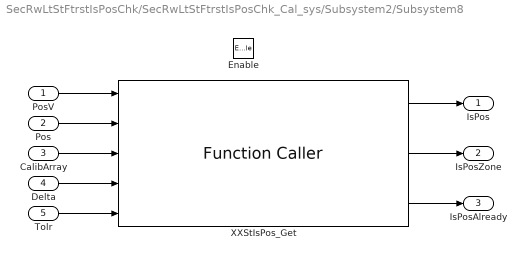
== system SecRwLtStFtrstIsPosChk/SecRwLtStFtrstIsPosChk_Cal_sys/Subsystem2/Subsystem8 ==
  PosV : Inport
  Pos : Inport  Port=2
  CalibArray : Inport  Port=3
  Delta : Inport  Port=4
  Tolr : Inport  Port=5
  Enable : EnablePort
  XXStIsPos_Get : FunctionCaller  FunctionPrototype=[IsPos,IsPosZone,IsPosAlready] = XXStIsPos_Get(PosV,Pos,CalibArray,Delta,Tolr)  InputArgumentSpecifications=boolean(true), uint16(1), uint16([1;1;1]), uint16(1), uint16(1)  OutputArgumentSpecifications=boolean(true), boolean(true), boolean(true)
  IsPos : Outport  VectorParamsAs1DForOutWhenUnconnected=off
  IsPosZone : Outport  Port=2  VectorParamsAs1DForOutWhenUnconnected=off
  IsPosAlready : Outport  Port=3  VectorParamsAs1DForOutWhenUnconnected=off
  wires:
  Delta/1 -> XXStIsPos_Get/4
  CalibArray/1 -> XXStIsPos_Get/3
  Tolr/1 -> XXStIsPos_Get/5
  PosV/1 -> XXStIsPos_Get/1
  XXStIsPos_Get/2 -> IsPosZone/1
  XXStIsPos_Get/3 -> IsPosAlready/1
  Pos/1 -> XXStIsPos_Get/2
  XXStIsPos_Get/1 -> IsPos/1
